simulink model "Noh_Nofusion"  (R2020b)
settings: Solver=FixedStepAuto  StartTime=0.0  StopTime=Inf  FixedStep=0.01  RelTol=1e-3
PostLoadFcn:
  | if any(exist('dsrtsu_mdlpostloadfcn', 'file') ~= 0), dsrtsu_mdlpostloadfcn('Execute', bdroot); end
InitFcn:
  | , if any(exist('rtifpga_mdlclblib', 'file') ~= 0), rtifpga_mdlclblib('Init', bdroot); end,
  | , if any(exist('dsmpb_private', 'file') ~= 0), dsmpb_private('dsmpb_mdlclblib', 'Init', bdroot); end,
undefined symbols (not defined in the file): ACC_TimeGap_DecSetSwt, ACC_TimeGap_IncSetSwt, AccelPedalPosn, AccelPedalPosnVldty, AccelPedlPosnDiagc, AccPedalOverride, ACU_ShiftInProgress, ADAS_Posn_CurLane, AESSwtReq, ALC_SwtReq, BrkPedalSts, CC_ACC_CANCEL_OFFSwt, CC_ACC_CRUISE_OFFSwt, CC_ACC_DecSetSpd_SetSwt, CC_ACC_IncSetSpd_ResuSwt, CC_ACCSwtErr, CharSpd_ms, CSA_NODE, CURRENT_GEAR, CurrentGearValid, DiscIntNeverNeededParam, DrvDoorSts, DrvSBR, DrvTrqReqOvld, ECMACCInterface, ECMRespACC, ELKSwtReq, EngLimpHomeSts, EngSpd, EngState, EngState_PHEV, EngTrqMaxActSpd, EngTrqMinAct, EPS_DrvInpTrqVal_HighReslolution, EPS_FailSts, EPS_LKATorqOvrlDlvd, EPS_LKATorqOvrlDlvdVld, EPS_LKATrqOvlDlvdSts, EPS_SteerMod, EPS_TrqSnsrSts, EQ4_APPINFO, EQ4_LA_ELEM, EQ4_LA_HDR, EQ4_LAP_ELEM, EQ4_LAP_HDR, EQ4_LH_ELEM, EQ4_LH_HDR, EQ4_LRE_ELEM, EQ4_LRE_HDR, ESS_PedSwtReq, ESS_VehSwtReq, FFogLmpSts_F_Pbox, FLWheelDriveDirection, FLWheelSpd, FrntWiprSwtSts, FrntWshrSwtSts, FRWheelDriveDirection, FRWheelSpd, HazardLmpSwtSts, HCU_AccelPedalPosn_Diag ... (+153)
libraries: simulink x132, dsmpblib x27
(part 2 of 14)

== system Noh_Nofusion/CAL ==
  Bus Assignment : BusAssignment  AssignedSignals=VehConfigHWA,VehConfigTJA,VehConfigLCK,VehConfigELK,VehConfigACC,VehConfigESS,VehConfigCC,VehConfigLKA,VehConfigLDW,VehConfigLCKIE,VehConfigiACC,VehConfigTSR,VehConfigAES
  Bus Assignment1 : BusAssignment  AssignedSignals=VehConfigADB,VehConfigHMA,VehConfigHMA_laser
  Bus Creator2 : BusCreator  Inputs=2
  Constant1 : Constant  Value=0  OutDataTypeStr=Bus: CAL_AHBC_CONFIG_BUS
  Constant2 : Constant  OutDataTypeStr=uint8
  Constant6 : Constant  Value=0  OutDataTypeStr=Bus: CAL_VSM_CONFIG_BUS
  Constant7 : Constant  OutDataTypeStr=uint8
  IfCALBus : Outport
  wires:
  Constant7/1 -> Bus Assignment/2, Bus Assignment/14, Bus Assignment/13, Bus Assignment/12, Bus Assignment/11, Bus Assignment/10, Bus Assignment/9, Bus Assignment/8, Bus Assignment/7, Bus Assignment/6, Bus Assignment/5, Bus Assignment/4, Bus Assignment/3
  Constant6/1 -> Bus Assignment/1
  Constant2/1 -> Bus Assignment1/4, Bus Assignment1/3, Bus Assignment1/2
  Bus Creator2/1 -> IfCALBus/1  "IfCALBus"
  Bus Assignment1/1 -> Bus Creator2/2  "CAL_AHBC_CONFIG"
  Bus Assignment/1 -> Bus Creator2/1  "CAL_VSM_CONFIG"
  Constant1/1 -> Bus Assignment1/1

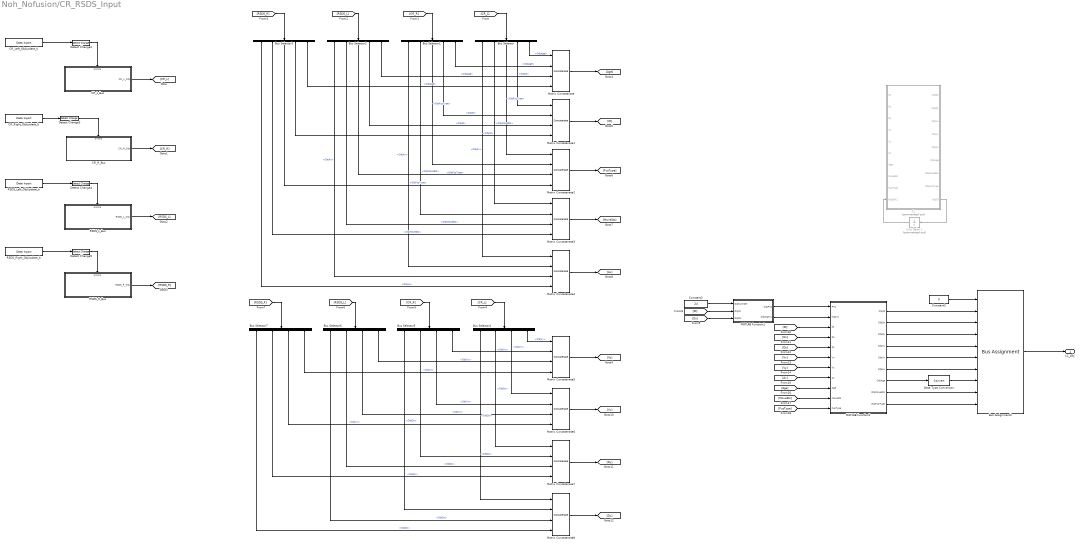
== system Noh_Nofusion/CR_RSDS_Input ==
  Bus Assignment3 : BusAssignment  AssignedSignals=Object_ID,Object_DX,Object_DY,Object_VX,Object_VY,Object_AX,Object_Age,Object_MovingState,Object_Fus_Type
  Bus Selector{,1..3} (4 alike) : BusSelector  OutputSignals=ObjAx,ObjMoveSts,ObjFusType,ObjID,ObjAge
  Bus Selector{4..7} (4 alike) : BusSelector  OutputSignals=ObjDx,ObjDy,ObjVx,ObjVy
  CL : MATLAB Function  Commented=on  TreatAsAtomicUnit=on
  CR_L_Bus : Subsystem
  CR_Left_ObjUpdate_b : dsmpblib/Data Inport  Priority=10000
      settings: SourceProductName=dSPACE Model Interface Blockset
  CR_R_Bus : Subsystem
  CR_Right_ObjUpdate_b : dsmpblib/Data Inport  Priority=10000
      settings: SourceProductName=dSPACE Model Interface Blockset
  Constant2 : Constant  Value=24  OutDataTypeStr=uint8
  Constant3 : Constant  Value=0  OutDataTypeStr=Bus: TOS_LC_BUS
  Data Type Conversion : DataTypeConversion
  Detect Change{2..5} (4 alike) : simulink/Logic and Bit Operations/Detect Change  vinit=0  OutDataTypeStr=boolean
  MATLAB Function1 : MATLAB Function  TreatAsAtomicUnit=on
  MATLAB Function2 : MATLAB Function  TreatAsAtomicUnit=on
  Matrix Concatenate{,1..8} (9 alike) : Concatenate  NumInputs=4
  RSDS_L_Bus : Subsystem
  RSDS_Left_ObjUpdate_b : dsmpblib/Data Inport  Priority=10000
      settings: SourceProductName=dSPACE Model Interface Blockset
  RSDS_R_Bus : Subsystem
  RSDS_Right_ObjUpdate_b : dsmpblib/Data Inport  Priority=10000
      settings: SourceProductName=dSPACE Model Interface Blockset
  Unit Delay1 : UnitDelay  Commented=on  SampleTime=-1  HasFrameUpgradeWarning=on
  LC_Obj : Outport  OutDataTypeStr=Bus: TOS_LC_BUS
  wires:
  Bus Selector5/4 -> Matrix Concatenate5/2  "<ObjVy>"
  [RSDS_L] -> Bus Selector2/1
  CR_Right_ObjUpdate_b/1 -> Detect Change3/1
  Matrix Concatenate8/1 -> [Dx]
  [CR_L] -> Bus Selector4/1
  Bus Selector3/5 -> Matrix Concatenate/4  "<ObjAge>"
  Bus Selector/4 -> Matrix Concatenate1/1  "<ObjID>"
  [RSDS_R] -> Bus Selector3/1
  RSDS_Left_ObjUpdate_b/1 -> Detect Change4/1
  [Vx] -> MATLAB Function2/6(Vx)
  Matrix Concatenate1/1 -> [ID]
  Bus Selector3/4 -> Matrix Concatenate1/4  "<ObjID>"
  Bus Selector1/5 -> Matrix Concatenate/2  "<ObjAge>"
  Bus Selector5/3 -> Matrix Concatenate6/2  "<ObjVx>"
  Bus Selector4/4 -> Matrix Concatenate5/1  "<ObjVy>"
  RSDS_Right_ObjUpdate_b/1 -> Detect Change5/1
  Bus Selector6/1 -> Matrix Concatenate8/3  "<ObjDx>"
  Bus Selector2/4 -> Matrix Concatenate1/3  "<ObjID>"
  Matrix Concatenate2/1 -> [FusType]
  Bus Selector7/2 -> Matrix Concatenate7/4  "<ObjDy>"
  Bus Selector2/2 -> Matrix Concatenate3/3  "<ObjMoveSts>"
  Bus Selector3/2 -> Matrix Concatenate3/4  "<ObjMoveSts>"
  Bus Selector4/1 -> Matrix Concatenate8/1  "<ObjDx>"
  Bus Selector6/2 -> Matrix Concatenate7/3  "<ObjDy>"
  Constant2/1 -> MATLAB Function1/1(ObjNumber)
  Constant3/1 -> Bus Assignment3/1
  [CR_R] -> Bus Selector5/1
  [RSDS_R] -> Bus Selector7/1
  [Dx] -> MATLAB Function2/4(Dx)
  [CR_R] -> Bus Selector1/1
  Bus Selector/5 -> Matrix Concatenate/1  "<ObjAge>"
  [FusType] -> MATLAB Function2/11(FusType)
  Bus Selector1/2 -> Matrix Concatenate3/2  "<ObjMoveSts>"
  CR_Left_ObjUpdate_b/1 -> Detect Change2/1
  Bus Selector6/4 -> Matrix Concatenate5/3  "<ObjVy>"
  Detect Change4/1 -> RSDS_L_Bus/Enable
  Detect Change5/1 -> RSDS_R_Bus/Enable
  Bus Selector/1 -> Matrix Concatenate4/1  "<ObjAx>"
  Detect Change2/1 -> CR_L_Bus/Enable
  Detect Change3/1 -> CR_R_Bus/Enable
  Bus Selector7/3 -> Matrix Concatenate6/4  "<ObjVx>"
  Bus Selector2/5 -> Matrix Concatenate/3  "<ObjAge>"
  Bus Selector3/1 -> Matrix Concatenate4/4  "<ObjAx>"
  Bus Selector7/4 -> Matrix Concatenate5/4  "<ObjVy>"
  [CR_L] -> Bus Selector/1
  MATLAB Function1/2(ObjMatrix) -> MATLAB Function2/2(Matrix)
  Bus Assignment3/1 -> LC_Obj/1
  Bus Selector6/3 -> Matrix Concatenate6/3  "<ObjVx>"
  Bus Selector2/3 -> Matrix Concatenate2/3  "<ObjFusType>"
  Matrix Concatenate3/1 -> [MoveSts]
  Matrix Concatenate7/1 -> [Dy]
  Bus Selector4/2 -> Matrix Concatenate7/1  "<ObjDy>"
  Matrix Concatenate5/1 -> [Vy]
  [Ax] -> MATLAB Function2/8(Ax)
  Bus Selector1/3 -> Matrix Concatenate2/2  "<ObjFusType>"
  Bus Selector2/1 -> Matrix Concatenate4/3  "<ObjAx>"
  [Vy] -> MATLAB Function2/7(Vy)
  Bus Selector3/3 -> Matrix Concatenate2/4  "<ObjFusType>"
  Bus Selector/3 -> Matrix Concatenate2/1  "<ObjFusType>"
  Bus Selector1/1 -> Matrix Concatenate4/2  "<ObjAx>"
  Bus Selector1/4 -> Matrix Concatenate1/2  "<ObjID>"
  Bus Selector5/2 -> Matrix Concatenate7/2  "<ObjDy>"
  [Dx] -> MATLAB Function1/3(ObjDx)
  [RSDS_L] -> Bus Selector6/1
  Bus Selector7/1 -> Matrix Concatenate8/4  "<ObjDx>"
  Bus Selector5/1 -> Matrix Concatenate8/2  "<ObjDx>"
  Bus Selector4/3 -> Matrix Concatenate6/1  "<ObjVx>"
  Bus Selector/2 -> Matrix Concatenate3/1  "<ObjMoveSts>"
  Matrix Concatenate6/1 -> [Vx]
  Matrix Concatenate4/1 -> [Ax]
  [ID] -> MATLAB Function1/2(ObjID)
  Matrix Concatenate/1 -> [Age]
  [Age] -> MATLAB Function2/9(Age)
  [Dy] -> MATLAB Function2/5(Dy)
  [MoveSts] -> MATLAB Function2/10(MoveSts)
  MATLAB Function1/1(ObjPrio) -> MATLAB Function2/1(Prio)
  [ID] -> MATLAB Function2/3(ID)
  RSDS_R_Bus/1(RSDS_R_Obj) -> [RSDS_R]
  RSDS_L_Bus/1(RSDS_L_Obj) -> [RSDS_L]
  CR_L_Bus/1(CR_L_Obj) -> [CR_L]
  CR_R_Bus/1(CR_R_Obj) -> [CR_R]
  CL/9(ObjID) -> Unit Delay1/1
  Unit Delay1/1 -> CL/10(ObjIDK1)
  MATLAB Function2/2(ObjDx) -> Bus Assignment3/3
  MATLAB Function2/1(ObjID) -> Bus Assignment3/2
  MATLAB Function2/3(ObjDy) -> Bus Assignment3/4
  MATLAB Function2/4(ObjVx) -> Bus Assignment3/5
  MATLAB Function2/5(ObjVy) -> Bus Assignment3/6
  MATLAB Function2/6(ObjAx) -> Bus Assignment3/7
  MATLAB Function2/7(ObjAge) -> Data Type Conversion/1
  MATLAB Function2/8(ObjMoveSts) -> Bus Assignment3/9
  MATLAB Function2/9(ObjFusType) -> Bus Assignment3/10
  Data Type Conversion/1 -> Bus Assignment3/8

== system Noh_Nofusion/Chassis1 ==
  note: DIAG-MON
      | (DiagnosticMonitor)
  note: HMI
      | (HumanMachineInterface)
  IfFaultTriggers : Inport
  IfFaultDTCs : Inport  Port=2
  IfVCANBus : Inport  Port=3  OutDataTypeStr=Bus: VCAN_BUS
  IfCALBus : Inport  Port=4
  IfVIEBus : Inport  Port=5
  IfVSMBus : Inport  Port=6
  IfLSMBus : Inport  Port=7
  IfLonCtrlBus : Inport  Port=8
  IfLatCtrlBus : Inport  Port=9
  IfPlanbus : Inport  Port=10
  IfVEQ4Bus : Inport  Port=11
  IfEHRBus : Inport  Port=12
  IfDMSBus : Inport  Port=13
  LaneBus : Inport  Port=14
  IfAEBBus : Inport  Port=15
  IfOSMBus : Inport  Port=16
  RoadBus : Inport  Port=17
  CSASim_IDC_L2_LampReq : Inport  Port=18
  function : TriggerPort  TriggerType=function-call  VariantControl=Variant
  Bus Assignment : BusAssignment  AssignedSignals=IFCAngCmdReqValue,IFCFuncAngCmdReqFlag,RollingCounter_IFC1,RollingCounter_IFC2
  Bus Assignment1 : BusAssignment  AssignedSignals=IFC_Line01_Dy,IFC_Line01_Curv,IFC_Line01_CurvChange,IFC_Line01_Type,IFC_Line02_Dy,IFC_Line02_Curv,IFC_Line02_CurvChange,IFC_Line02_Type,IFC_Line03_Dy,IFC_Line03_Curv,IFC_Line03_CurvChange,IFC_Line03_Type,IFC_Line04_Dy,IFC_Line04_Curv,IFC_Line04_CurvChange,IFC_Line04_Type,IFC_Roadedge01_Dy,IFC_Roadedge01_Curv,IFC_Roadedge01_CurvChange,IFC_Roadedge01_Type,IFC_Roadedge02_Dy,IFC_Roadedge02_Curv,IFC_Roadedge02_CurvChange,IFC_Roadedge02_Type
  Bus Assignment2 : BusAssignment  AssignedSignals=IFC_Line01_HeadingAngle,IFC_Line02_HeadingAngle,IFC_Line03_HeadingAngle,IFC_Line04_HeadingAngle,IFC_Roadedge01_HeadingAngle,IFC_Roadedge02_HeadingAngle
  Bus Assignment3 : BusAssignment  AssignedSignals=ACCTgtObjAx,ACCTgtObjAy,ACCTgtObjCntAlive,ACCTgtObjDx,ACCTgtObjDy,ACCTgtObjExist,ACCTgtObjID,ACCTgtObjObstcl,ACCTgtObjState,ACCTgtObjVideoCfmd,ACCTgtObjVx,ACCTgtObjVy,ACC_SOSReq,BrdgDst,CurveDst,DrvgOnHiWay,DrvgOnRiLane,DrvrSts,HandsoffDetd,MapDataValid,NavSpdLimUnit,RampDst,RoadCrvt,RoadCrvtFar,SpdLimit,SpdLimitDst,TunnelDst
  Bus Assignment4 : BusAssignment  AssignedSignals=Longctrl_DecelToStopReq,Longctrl_Decel_Req,Longctrl_Decel_ReqValue,Longctrl_EngTrqReq,Longctrl_EngTrqReqActive,Longctrl_HCUTrqReq,Longctrl_HCUTrqReqActive,ACC_CRInterface,ActualTargetSpeed,Longctrl_DrvOFF_Req,Longctrl_FuelCutOffPrevn,Longctrl_ModSts,Longctrl_ParkShiftReq,Longctrl_VehHldReq,HWP_TgtAccel_L2,RollingCounter_ACC1,RollingCounter_ACC2,RollingCounter_ACC10
  Bus Assignment5 : BusAssignment  AssignedSignals=ACC_EgoStatus,ACC_FctSts,ACC_InterSysInfoDisp,ACC_LeTargrtDection,ACC_LeTargrt_02_Detn,ACC_LeTgtDx,ACC_LeTgtDy,ACC_LeTgtHeading,ACC_LeTgtObjBarDisp,ACC_LeTgtTyp,ACC_LeTgt_02_Dx,ACC_LeTgt_02_Dy,ACC_LeTgt_02_Typ,ACC_LeTgtfusion,ACC_ModDisp,ACC_ObjDetecte,ACC_PotentialTgtDetn,ACC_PotentialTgtDx,ACC_PotentialTgtDy,ACC_PotentialTgtHeading,ACC_PotentialTgtTyp,ACC_PotentialTgtfusion,ACC_RiTargrtDetn,ACC_RiTargrt_02_Detn,ACC_RiTgtDx,ACC_RiTgtDy,ACC_RiTgtHeading,ACC_RiTgtObjBarDisp,ACC_RiTgtTyp,ACC_RiTgt_02_Dx,ACC_RiTgt_02_Dy,ACC_RiTgt_02_Typ,ACC_RiTgtfusion,ACC_RlvTgtDetn,ACC_RlvTgtDx,ACC_RlvTgtDy,ACC_RlvTgtHeading,ACC_RlvTgtTyp,ACC_RlvTgtfusion,ACC_SpdSetValue,ACC_TakeOverReq,ACC_TgtObjBarDisp,ACC_TimeGapSet,ADAS_DriverInloop_Monitor,ALC_InterSysInfoDisp,ALC_Resp,CruCha_ModDisp,CruChar_InterSysInfoDisp,HWA_InterSysInfoDisp,HWA_LaneChange,HWA_LaneChangeReq,HWA_ModDisp,HWA_Resp,HWA_SnvtySet_Resp,HWA_warning,ICA_HandsOffResp,ISL_InterSysInfoDisp,ISL_Resp,IntelligentCurveAct,Request_driveoff,TJA_ACC_SelSts,TJA_ICA_InterSysInfoDisp,TJA_ICA_ModDisp,RollingCounter_ACC3,RollingCounter_ACC4,RollingCounter_ACC8,RollingCounter_ACC6,RollingCounter_ACC7
  Bus Assignment6 : BusAssignment  AssignedSignals=AESErrSts,AESResp,AESSts,AESintervention,CameraBlockageSts,ELKMainState,ELKResp,ESSErrSts,ESSSts,ESS_PedResp,ESS_VehResp,ESSintervention,IFCCalibrationSts,IFCHUTInterface,IFC_Handsoffwarn,IFC_LaneCurve,IFC_LeLaneTyp,IFC_LeLane_dy,IFC_NextLeLaneTyp,IFC_NextLeLane_dy,IFC_NextRiLaneTyp,IFC_NextRiLane_dy,IFC_RiLaneTyp,IFC_RiLane_dy,IntelligentEvaResp,LCKResp,LDWResp,LDW_LKAWarn,LDW_LKA_Snvty,LKAResp,LSSErrSts,LSSFuncSts,LSSIntervention,LSSResp,LSSWarnFormResp,LaneAvailability,TJA_FollowSts,RollingCounter_IFC3,RollingCounter_IFC4,RollingCounter_IFC5,RollingCounter_IFC6
  Bus Assignment7 : BusAssignment  AssignedSignals=IDC_L2_EmgyLightReq,IDC_L2_FWiperReq,IDC_L2_TurnLightReq,RollingCounter_IFC7
  Bus Selector : BusSelector  OutputSignals=LONC_CTRL_OUT.Longctrl_Decel_Req,LONC_CTRL_OUT.Longctrl_Decel_ReqValue,LONC_CTRL_OUT.Longctrl_EngTrqReq,LONC_CTRL_OUT.Longctrl_EngTrqReqActive,LONC_Hybrid_CTRL_OUT.Longctrl_HCUTrqReq,LONC_Hybrid_CTRL_OUT.Longctrl_HCUTrqReqActive
  Bus Selector1 : BusSelector  OutputSignals=LATC_IFCAngCmdReqValue,LATC_IFCFuncAngCmdReqFlag
  Bus Selector10 : BusSelector  OutputSignals=HMI_ACC_FD4.ACCTgtObjAx,HMI_ACC_FD4.ACCTgtObjAy,HMI_ACC_FD4.ACCTgtObjCntAlive,HMI_ACC_FD4.ACCTgtObjDx,HMI_ACC_FD4.ACCTgtObjDy,HMI_ACC_FD4.ACCTgtObjExist,HMI_ACC_FD4.ACCTgtObjID,HMI_ACC_FD4.ACCTgtObjObstcl,HMI_ACC_FD4.ACCTgtObjState,HMI_ACC_FD4.ACCTgtObjVideoCfmd,HMI_ACC_FD4.ACCTgtObjVx,HMI_ACC_FD4.ACCTgtObjVy,HMI_ACC_FD4.ACC_SOSReq,HMI_ACC_FD4.BrdgDst,HMI_ACC_FD4.CurveDst,HMI_ACC_FD4.DrvgOnHiWay,HMI_ACC_FD4.DrvgOnRiLane,HMI_ACC_FD4.DrvrSts,HMI_ACC_FD4.HandsoffDetd,HMI_ACC_FD4.MapDataValid,HMI_ACC_FD4.NavSpdLimUnit,HMI_ACC_FD4.RampDst,HMI_ACC_FD4.RoadCrvt,HMI_ACC_FD4.RoadCrvtFar,HMI_ACC_FD4.SpdLimit,HMI_ACC_FD4.SpdLimitDst,HMI_ACC_FD4.TunnelDst
  Bus Selector18 : BusSelector  OutputSignals=PLAN_Longctrl_DecelToStopReq
  Bus Selector19 : BusSelector  OutputSignals=HMI_IFC_FD3.IDC_L2_EmgyLightReq,HMI_IFC_FD3.IDC_L2_FWiperReq
  Bus Selector2 : BusSelector  OutputSignals=HMI_ACC_FD1.ACC_CRInterface,HMI_ACC_FD1.ActualTargetSpeed,HMI_ACC_FD1.Longctrl_DrvOFF_Req,HMI_ACC_FD1.Longctrl_FuelCutOffPrevn,HMI_ACC_FD1.Longctrl_ModSts,HMI_ACC_FD1.Longctrl_ParkShiftReq,HMI_ACC_FD1.Longctrl_VehHldReq
  Bus Selector3 : BusSelector  OutputSignals=AESErrSts,HMI_IFC_FD2.AESResp,HMI_IFC_FD2.AESSts,HMI_IFC_FD2.AESintervention,HMI_IFC_FD2.CameraBlockageSts,HMI_IFC_FD2.ELKMainState,HMI_IFC_FD2.ELKResp,ESSErrSts,HMI_IFC_FD2.ESSSts,HMI_IFC_FD2.ESS_PedResp,HMI_IFC_FD2.ESS_VehResp,HMI_IFC_FD2.ESSintervention,HMI_IFC_FD2.IFCCalibrationSts,HMI_IFC_FD2.IFCHUTInterface,HMI_IFC_FD2.IFC_Handsoffwarn,HMI_IFC_FD2.IFC_LaneCurve,HMI_IFC_FD2.IFC_LeLaneTyp,HMI_IFC_FD2.IFC_LeLane_dy,HMI_IFC_FD2.IFC_NextLeLaneTyp,HMI_IFC_FD2.IFC_NextLeLane_dy,HMI_IFC_FD2.IFC_NextRiLaneTyp,HMI_IFC_FD2.IFC_NextRiLane_dy,HMI_IFC_FD2.IFC_RiLaneTyp,HMI_IFC_FD2.IFC_RiLane_dy,HMI_IFC_FD2.IntelligentEvaResp,HMI_IFC_FD2.LCKResp,HMI_IFC_FD2.LDWResp,HMI_IFC_FD2.LDW_LKAWarn,HMI_IFC_FD2.LDW_LKA_Snvty,HMI_IFC_FD2.LKAResp,HMI_IFC_FD2.LSSErrSts,HMI_IFC_FD2.LSSFuncSts,HMI_IFC_FD2.LSSIntervention,HMI_IFC_FD2.LSSResp,HMI_IFC_FD2.LSSWarnFormResp,HMI_IFC_FD2.LaneAvailability,HMI_IFC_FD2.TJA_FollowSts
  Bus Selector5 : BusSelector  OutputSignals=HMI_IFC_FD5.IFC_Line01_Dy,HMI_IFC_FD5.IFC_Line01_Curv,HMI_IFC_FD5.IFC_Line01_CurvChange,HMI_IFC_FD5.IFC_Line01_Type,HMI_IFC_FD5.IFC_Line02_Dy,HMI_IFC_FD5.IFC_Line02_Curv,HMI_IFC_FD5.IFC_Line02_CurvChange,HMI_IFC_FD5.IFC_Line02_Type,HMI_IFC_FD5.IFC_Line03_Dy,HMI_IFC_FD5.IFC_Line03_Curv,HMI_IFC_FD5.IFC_Line03_CurvChange,HMI_IFC_FD5.IFC_Line03_Type,HMI_IFC_FD5.IFC_Line04_Dy,HMI_IFC_FD5.IFC_Line04_Curv,HMI_IFC_FD5.IFC_Line04_CurvChange,HMI_IFC_FD5.IFC_Line04_Type,HMI_IFC_FD5.IFC_Roadedge01_Dy,HMI_IFC_FD5.IFC_Roadedge01_Curv,HMI_IFC_FD5.IFC_Roadedge01_CurvChange,HMI_IFC_FD5.IFC_Roadedge01_Type,HMI_IFC_FD5.IFC_Roadedge02_Dy,HMI_IFC_FD5.IFC_Roadedge02_Curv,HMI_IFC_FD5.IFC_Roadedge02_CurvChange,HMI_IFC_FD5.IFC_Roadedge02_Type
  Bus Selector6 : BusSelector  OutputSignals=HMI_IFC_FD6.IFC_Line01_HeadingAngle,HMI_IFC_FD6.IFC_Line02_HeadingAngle,HMI_IFC_FD6.IFC_Line03_HeadingAngle,HMI_IFC_FD6.IFC_Line04_HeadingAngle,HMI_IFC_FD6.IFC_Roadedge01_HeadingAngle,HMI_IFC_FD6.IFC_Roadedge02_HeadingAngle
  Bus Selector8 : BusSelector  OutputSignals=HMI_ACC_FD2.ACC_EgoStatus,HMI_ACC_FD2.ACC_FctSts,HMI_ACC_FD2.ACC_InterSysInfoDisp,HMI_ACC_FD2.ACC_LeTargrtDection,HMI_ACC_FD2.ACC_LeTargrt_02_Detn,HMI_ACC_FD2.ACC_LeTgtDx,HMI_ACC_FD2.ACC_LeTgtDy,HMI_ACC_FD2.ACC_LeTgtHeading,HMI_ACC_FD2.ACC_LeTgtObjBarDisp,HMI_ACC_FD2.ACC_LeTgtTyp,HMI_ACC_FD2.ACC_LeTgt_02_Dy,HMI_ACC_FD2.ACC_LeTgt_02_Dx,HMI_ACC_FD2.ACC_LeTgt_02_Typ,HMI_ACC_FD2.ACC_LeTgtfusion,HMI_ACC_FD2.ACC_ModDisp,HMI_ACC_FD2.ACC_ObjDetecte,HMI_ACC_FD2.ACC_PotentialTgtDetn,HMI_ACC_FD2.ACC_PotentialTgtDx,HMI_ACC_FD2.ACC_PotentialTgtDy,HMI_ACC_FD2.ACC_PotentialTgtHeading,HMI_ACC_FD2.ACC_PotentialTgtTyp,HMI_ACC_FD2.ACC_PotentialTgtfusion,HMI_ACC_FD2.ACC_RiTargrtDetn,HMI_ACC_FD2.ACC_RiTargrt_02_Detn,HMI_ACC_FD2.ACC_RiTgtDx,HMI_ACC_FD2.ACC_RiTgtDy,HMI_ACC_FD2.ACC_RiTgtHeading,HMI_ACC_FD2.ACC_RiTgtObjBarDisp,HMI_ACC_FD2.ACC_RiTgtTyp,HMI_ACC_FD2.ACC_RiTgt_02_Dx,HMI_ACC_FD2.ACC_RiTgt_02_Dy,HMI_ACC_FD2.ACC_RiTgt_02_Typ,HMI_ACC_FD2.ACC_RiTgtfusion,HMI_ACC_FD2.ACC_RlvTgtDetn,HMI_ACC_FD2.ACC_RlvTgtDx,HMI_ACC_FD2.ACC_RlvTgtDy,HMI_ACC_FD2.ACC_RlvTgtHeading,HMI_ACC_FD2.ACC_RlvTgtTyp,HMI_ACC_FD2.ACC_RlvTgtfusion,HMI_ACC_FD2.ACC_SpdSetValue,HMI_ACC_FD2.ACC_TakeOverReq,HMI_ACC_FD2.ACC_TgtObjBarDisp,HMI_ACC_FD2.ACC_TimeGapSet,HMI_ACC_FD2.ADAS_DriverInloop_Monitor,HMI_ACC_FD2.ALC_InterSysInfoDisp,HMI_ACC_FD2.ALC_Resp,HMI_ACC_FD2.CruCha_ModDisp,HMI_ACC_FD2.CruChar_InterSysInfoDisp,HMI_ACC_FD2.HWA_InterSysInfoDisp,HMI_ACC_FD2.HWA_LaneChange,HMI_ACC_FD2.HWA_LaneChangeReq,HMI_ACC_FD2.HWA_ModDisp,HMI_ACC_FD2.HWA_Resp,HMI_ACC_FD2.HWA_SnvtySet_Resp,HMI_ACC_FD2.HWA_warning,HMI_ACC_FD2.ICA_HandsOffResp,HMI_ACC_FD2.ISL_InterSysInfoDisp,HMI_ACC_FD2.ISL_Resp,HMI_ACC_FD2.IntelligentCurveAct,HMI_ACC_FD2.Request_driveoff,HMI_ACC_FD2.TJA_ACC_SelSts,HMI_ACC_FD2.TJA_ICA_InterSysInfoDisp,HMI_ACC_FD2.TJA_ICA_ModDisp
  Constant : Constant  Value=0  OutDataTypeStr=Bus: IFC_FD1_MSG_BUS
  Constant10 : Constant  Value=0  OutDataTypeStr=Bus: ACC_FD2_MSG_BUS
  Constant12 : Constant  Value=0  OutDataTypeStr=Bus: IFC_FD3_MSG_BUS
  Constant3 : Constant  Value=0  OutDataTypeStr=Bus: IFC_FD2_MSG_BUS
  Constant5 : Constant  Value=0  OutDataTypeStr=Bus: IFC_FD5_MSG_BUS
  Constant6 : Constant  Value=0  OutDataTypeStr=Bus: IFC_FD6_MSG_BUS
  Constant7 : Constant  Value=0  OutDataTypeStr=Bus: ACC_FD4_MSG_BUS
  Constant8 : Constant  Value=0  OutDataTypeStr=Bus: ACC_FD1_MSG_BUS
  Constant9 : Constant  Value=127  OutDataTypeStr=int8
  Counter Limited{,1..4} (5 alike) : simulink/Sources/Counter Limited  uplimit=15  tsamp=-1
  HMA : Subsystem  Commented=on
  HMI : Subsystem
  IfPlanbus1 : InportShadow  Port=10
  IFC_FD1 : Outport
  IFC_FD2 : Outport  Port=2
  IFC_FD3 : Outport  Port=3
  IFC_FD5 : Outport  Port=4
  IFC_FD6 : Outport  Port=5
  ACC_FD1 : Outport  Port=6
  ACC_FD2 : Outport  Port=7
  ACC_FD4 : Outport  Port=8
  wires:
  IfVCANBus/1 -> HMI/1(IfVCANBus), HMA/1(IfCANBus)
  IfVEQ4Bus/1 -> HMA/4(IfEQ4Bus)
  IfCALBus/1 -> HMA/2(IfCALBus)
  IfFaultTriggers/1 -> HMA/3(IfDIAGBus), HMI/2(IfFaultTriggers)
  IfLonCtrlBus/1 -> [IfLonCtrlBus], HMI/5(IfLonCtrlBus)  "IfLonCtrlBus"
  IfOSMBus/1 -> HMI/6(IfOSMBus)
  IfAEBBus/1 -> HMI/7(IfAEBBus)
  IfEHRBus/1 -> HMI/8(IfEHRBus)
  IfDMSBus/1 -> HMI/9(IfDMSBus)
  LaneBus/1 -> HMI/10(LaneBus)
  RoadBus/1 -> HMI/11(RoadBus)
  HMI/1(IfHMIBus) -> Bus Selector2/1, Bus Selector10/1, Bus Selector8/1, Bus Selector6/1, Bus Selector5/1, Bus Selector19/1, Bus Selector3/1  "HMI"
  IfVSMBus/1 -> [IfVSMBus], HMI/4(IfVSMBus)
  Bus Assignment3/1 -> ACC_FD4/1
  Bus Assignment4/1 -> ACC_FD1/1
  IfPlanbus/1 -> HMI/3(IfPlanbus)
  IfPlanbus1/1 -> Bus Selector18/1
  Bus Selector18/1 -> Bus Assignment4/2  "<PLAN_Longctrl_DecelToStopReq>"
  Bus Selector1/1 -> Bus Assignment/2  "<LATC_IFCAngCmdReqValue>"
  Bus Selector1/2 -> Bus Assignment/3  "<LATC_IFCFuncAngCmdReqFlag>"
  IfLatCtrlBus/1 -> Bus Selector1/1
  Constant/1 -> Bus Assignment/1
  Bus Assignment/1 -> IFC_FD1/1
  Constant5/1 -> Bus Assignment1/1
  Bus Selector5/1 -> Bus Assignment1/2  "<IFC_Line01_Dy>"
  Bus Selector5/2 -> Bus Assignment1/3  "<IFC_Line01_Curv>"
  Bus Selector5/3 -> Bus Assignment1/4  "<IFC_Line01_CurvChange>"
  Bus Selector5/4 -> Bus Assignment1/5  "<IFC_Line01_Type>"
  Bus Selector5/5 -> Bus Assignment1/6  "<IFC_Line02_Dy>"
  Bus Selector5/6 -> Bus Assignment1/7  "<IFC_Line02_Curv>"
  Bus Selector5/7 -> Bus Assignment1/8  "<IFC_Line02_CurvChange>"
  Bus Selector5/8 -> Bus Assignment1/9  "<IFC_Line02_Type>"
  Bus Selector5/9 -> Bus Assignment1/10  "<IFC_Line03_Dy>"
  Bus Selector5/10 -> Bus Assignment1/11  "<IFC_Line03_Curv>"
  Bus Selector5/11 -> Bus Assignment1/12  "<IFC_Line03_CurvChange>"
  Bus Selector5/12 -> Bus Assignment1/13  "<IFC_Line03_Type>"
  Bus Selector5/13 -> Bus Assignment1/14  "<IFC_Line04_Dy>"
  Bus Selector5/14 -> Bus Assignment1/15  "<IFC_Line04_Curv>"
  Bus Selector5/15 -> Bus Assignment1/16  "<IFC_Line04_CurvChange>"
  Bus Selector5/16 -> Bus Assignment1/17  "<IFC_Line04_Type>"
  Bus Selector5/17 -> Bus Assignment1/18  "<IFC_Roadedge01_Dy>"
  Bus Selector5/18 -> Bus Assignment1/19  "<IFC_Roadedge01_Curv>"
  Bus Selector5/19 -> Bus Assignment1/20  "<IFC_Roadedge01_CurvChange>"
  Bus Selector5/20 -> Bus Assignment1/21  "<IFC_Roadedge01_Type>"
  Bus Selector5/21 -> Bus Assignment1/22  "<IFC_Roadedge02_Dy>"
  Bus Selector5/22 -> Bus Assignment1/23  "<IFC_Roadedge02_Curv>"
  Bus Selector5/23 -> Bus Assignment1/24  "<IFC_Roadedge02_CurvChange>"
  Bus Selector5/24 -> Bus Assignment1/25  "<IFC_Roadedge02_Type>"
  Bus Assignment1/1 -> IFC_FD5/1
  Constant6/1 -> Bus Assignment2/1
  Bus Selector6/6 -> Bus Assignment2/7  "<IFC_Roadedge02_HeadingAngle>"
  Bus Selector6/5 -> Bus Assignment2/6  "<IFC_Roadedge01_HeadingAngle>"
  Bus Selector6/4 -> Bus Assignment2/5  "<IFC_Line04_HeadingAngle>"
  Bus Selector6/3 -> Bus Assignment2/4  "<IFC_Line03_HeadingAngle>"
  Bus Selector6/2 -> Bus Assignment2/3  "<IFC_Line02_HeadingAngle>"
  Bus Selector6/1 -> Bus Assignment2/2  "<IFC_Line01_HeadingAngle>"
  Bus Assignment2/1 -> IFC_FD6/1
  Constant7/1 -> Bus Assignment3/1
  Bus Selector10/1 -> Bus Assignment3/2  "<ACCTgtObjAx>"
  Bus Selector10/2 -> Bus Assignment3/3  "<ACCTgtObjAy>"
  Bus Selector10/3 -> Bus Assignment3/4  "<ACCTgtObjCntAlive>"
  Bus Selector10/4 -> Bus Assignment3/5  "<ACCTgtObjDx>"
  Bus Selector10/5 -> Bus Assignment3/6  "<ACCTgtObjDy>"
  Bus Selector10/6 -> Bus Assignment3/7  "<ACCTgtObjExist>"
  Bus Selector10/7 -> Bus Assignment3/8  "<ACCTgtObjID>"
  Bus Selector10/8 -> Bus Assignment3/9  "<ACCTgtObjObstcl>"
  Bus Selector10/9 -> Bus Assignment3/10  "<ACCTgtObjState>"
  Bus Selector10/10 -> Bus Assignment3/11  "<ACCTgtObjVideoCfmd>"
  Bus Selector10/11 -> Bus Assignment3/12  "<ACCTgtObjVx>"
  Bus Selector10/12 -> Bus Assignment3/13  "<ACCTgtObjVy>"
  Bus Selector10/13 -> Bus Assignment3/14  "<ACC_SOSReq>"
  Bus Selector10/14 -> Bus Assignment3/15  "<BrdgDst>"
  Bus Selector10/15 -> Bus Assignment3/16  "<CurveDst>"
  Bus Selector10/16 -> Bus Assignment3/17  "<DrvgOnHiWay>"
  Bus Selector10/17 -> Bus Assignment3/18  "<DrvgOnRiLane>"
  Bus Selector10/18 -> Bus Assignment3/19  "<DrvrSts>"
  Bus Selector10/19 -> Bus Assignment3/20  "<HandsoffDetd>"
  Bus Selector10/20 -> Bus Assignment3/21  "<MapDataValid>"
  Bus Selector10/21 -> Bus Assignment3/22  "<NavSpdLimUnit>"
  Bus Selector10/22 -> Bus Assignment3/23  "<RampDst>"
  Bus Selector10/23 -> Bus Assignment3/24  "<RoadCrvt>"
  Bus Selector10/24 -> Bus Assignment3/25  "<RoadCrvtFar>"
  Bus Selector10/25 -> Bus Assignment3/26  "<SpdLimit>"
  Bus Selector10/26 -> Bus Assignment3/27  "<SpdLimitDst>"
  Bus Selector10/27 -> Bus Assignment3/28  "<TunnelDst>"
  Constant9/1 -> Bus Assignment4/16
  Bus Selector2/7 -> Bus Assignment4/15  "<Longctrl_VehHldReq>"
  Bus Selector2/6 -> Bus Assignment4/14  "<Longctrl_ParkShiftReq>"
  Bus Selector2/5 -> Bus Assignment4/13  "<Longctrl_ModSts>"
  Bus Selector2/4 -> Bus Assignment4/12  "<Longctrl_FuelCutOffPrevn>"
  Bus Selector2/3 -> Bus Assignment4/11  "<Longctrl_DrvOFF_Req>"
  Bus Selector2/2 -> Bus Assignment4/10  "<ActualTargetSpeed>"
  Bus Selector2/1 -> Bus Assignment4/9  "<ACC_CRInterface>"
  Constant8/1 -> Bus Assignment4/1
  Counter Limited/1 -> Bus Assignment4/18, Bus Assignment4/17, Bus Assignment4/19
  [IfLonCtrlBus] -> Bus Selector/1
  Bus Selector/3 -> Bus Assignment4/5  "<Longctrl_EngTrqReq>"
  Bus Selector/2 -> Bus Assignment4/4  "<Longctrl_Decel_ReqValue>"
  Bus Selector/4 -> Bus Assignment4/6  "<Longctrl_EngTrqReqActive>"
  Bus Selector/1 -> Bus Assignment4/3  "<Longctrl_Decel_Req>"
  Bus Selector/5 -> Bus Assignment4/7  "<Longctrl_HCUTrqReq>"
  Bus Selector/6 -> Bus Assignment4/8  "<Longctrl_HCUTrqReqActive>"
  Constant10/1 -> Bus Assignment5/1
  Bus Selector8/1 -> Bus Assignment5/2  "<ACC_EgoStatus>"
  Bus Selector8/2 -> Bus Assignment5/3  "<ACC_FctSts>"
  Bus Selector8/3 -> Bus Assignment5/4  "<ACC_InterSysInfoDisp>"
  Bus Selector8/4 -> Bus Assignment5/5  "<ACC_LeTargrtDection>"
  Bus Selector8/5 -> Bus Assignment5/6  "<ACC_LeTargrt_02_Detn>"
  Bus Selector8/6 -> Bus Assignment5/7  "<ACC_LeTgtDx>"
  Bus Selector8/7 -> Bus Assignment5/8  "<ACC_LeTgtDy>"
  Bus Selector8/8 -> Bus Assignment5/9  "<ACC_LeTgtHeading>"
  Bus Selector8/9 -> Bus Assignment5/10  "<ACC_LeTgtObjBarDisp>"
  Bus Selector8/10 -> Bus Assignment5/11  "<ACC_LeTgtTyp>"
  Bus Selector8/11 -> Bus Assignment5/12  "<ACC_LeTgt_02_Dy>"
  Bus Selector8/12 -> Bus Assignment5/13  "<ACC_LeTgt_02_Dx>"
  Bus Selector8/13 -> Bus Assignment5/14  "<ACC_LeTgt_02_Typ>"
  Bus Selector8/14 -> Bus Assignment5/15  "<ACC_LeTgtfusion>"
  Bus Selector8/15 -> Bus Assignment5/16  "<ACC_ModDisp>"
  Bus Selector8/16 -> Bus Assignment5/17  "<ACC_ObjDetecte>"
  Bus Selector8/17 -> Bus Assignment5/18  "<ACC_PotentialTgtDetn>"
  Bus Selector8/18 -> Bus Assignment5/19  "<ACC_PotentialTgtDx>"
  Bus Selector8/19 -> Bus Assignment5/20  "<ACC_PotentialTgtDy>"
  Bus Selector8/20 -> Bus Assignment5/21  "<ACC_PotentialTgtHeading>"
  Bus Selector8/21 -> Bus Assignment5/22  "<ACC_PotentialTgtTyp>"
  Bus Selector8/22 -> Bus Assignment5/23  "<ACC_PotentialTgtfusion>"
  Bus Selector8/23 -> Bus Assignment5/24  "<ACC_RiTargrtDetn>"
  Bus Selector8/24 -> Bus Assignment5/25  "<ACC_RiTargrt_02_Detn>"
  Bus Selector8/25 -> Bus Assignment5/26  "<ACC_RiTgtDx>"
  Bus Selector8/26 -> Bus Assignment5/27  "<ACC_RiTgtDy>"
  Bus Selector8/27 -> Bus Assignment5/28  "<ACC_RiTgtHeading>"
  Bus Selector8/28 -> Bus Assignment5/29  "<ACC_RiTgtObjBarDisp>"
  Bus Selector8/29 -> Bus Assignment5/30  "<ACC_RiTgtTyp>"
  Bus Selector8/30 -> Bus Assignment5/31  "<ACC_RiTgt_02_Dx>"
  Bus Selector8/31 -> Bus Assignment5/32  "<ACC_RiTgt_02_Dy>"
  Bus Selector8/32 -> Bus Assignment5/33  "<ACC_RiTgt_02_Typ>"
  Bus Selector8/33 -> Bus Assignment5/34  "<ACC_RiTgtfusion>"
  Bus Selector8/34 -> Bus Assignment5/35  "<ACC_RlvTgtDetn>"
  Bus Selector8/35 -> Bus Assignment5/36  "<ACC_RlvTgtDx>"
  Bus Selector8/36 -> Bus Assignment5/37  "<ACC_RlvTgtDy>"
  Bus Selector8/37 -> Bus Assignment5/38  "<ACC_RlvTgtHeading>"
  Bus Selector8/38 -> Bus Assignment5/39  "<ACC_RlvTgtTyp>"
  Bus Selector8/39 -> Bus Assignment5/40  "<ACC_RlvTgtfusion>"
  Bus Selector8/40 -> Bus Assignment5/41  "<ACC_SpdSetValue>"
  Bus Selector8/41 -> Bus Assignment5/42  "<ACC_TakeOverReq>"
  Bus Selector8/42 -> Bus Assignment5/43  "<ACC_TgtObjBarDisp>"
  Bus Selector8/43 -> Bus Assignment5/44  "<ACC_TimeGapSet>"
  Bus Selector8/44 -> Bus Assignment5/45  "<ADAS_DriverInloop_Monitor>"
  Bus Selector8/45 -> Bus Assignment5/46  "<ALC_InterSysInfoDisp>"
  Bus Selector8/46 -> Bus Assignment5/47  "<ALC_Resp>"
  Bus Selector8/47 -> Bus Assignment5/48  "<CruCha_ModDisp>"
  Bus Selector8/48 -> Bus Assignment5/49  "<CruChar_InterSysInfoDisp>"
  Bus Selector8/49 -> Bus Assignment5/50  "<HWA_InterSysInfoDisp>"
  Bus Selector8/50 -> Bus Assignment5/51  "<HWA_LaneChange>"
  Bus Selector8/51 -> Bus Assignment5/52  "<HWA_LaneChangeReq>"
  Bus Selector8/52 -> Bus Assignment5/53  "<HWA_ModDisp>"
  Bus Selector8/53 -> Bus Assignment5/54  "<HWA_Resp>"
  Bus Selector8/54 -> Bus Assignment5/55  "<HWA_SnvtySet_Resp>"
  Bus Selector8/55 -> Bus Assignment5/56  "<HWA_warning>"
  Bus Selector8/56 -> Bus Assignment5/57  "<ICA_HandsOffResp>"
  Bus Selector8/57 -> Bus Assignment5/58  "<ISL_InterSysInfoDisp>"
  Bus Selector8/58 -> Bus Assignment5/59  "<ISL_Resp>"
  Bus Selector8/59 -> Bus Assignment5/60  "<IntelligentCurveAct>"
  Counter Limited1/1 -> Bus Assignment5/68, Bus Assignment5/65, Bus Assignment5/66, Bus Assignment5/67, Bus Assignment5/69
  Bus Selector8/60 -> Bus Assignment5/61  "<Request_driveoff>"
  Bus Selector8/61 -> Bus Assignment5/62  "<TJA_ACC_SelSts>"
  Bus Selector8/62 -> Bus Assignment5/63  "<TJA_ICA_InterSysInfoDisp>"
  Bus Selector8/63 -> Bus Assignment5/64  "<TJA_ICA_ModDisp>"
  Bus Assignment5/1 -> ACC_FD2/1
  Constant3/1 -> Bus Assignment6/1
  Bus Selector3/1 -> Bus Assignment6/2  "<AESErrSts>"
  Bus Selector3/2 -> Bus Assignment6/3  "<AESResp>"
  Bus Selector3/3 -> Bus Assignment6/4  "<AESSts>"
  Bus Selector3/4 -> Bus Assignment6/5  "<AESintervention>"
  Bus Selector3/5 -> Bus Assignment6/6  "<CameraBlockageSts>"
  Bus Selector3/6 -> Bus Assignment6/7  "<ELKMainState>"
  Bus Selector3/7 -> Bus Assignment6/8  "<ELKResp>"
  Bus Selector3/8 -> Bus Assignment6/9  "<ESSErrSts>"
  Bus Selector3/9 -> Bus Assignment6/10  "<ESSSts>"
  Bus Selector3/10 -> Bus Assignment6/11  "<ESS_PedResp>"
  Bus Selector3/11 -> Bus Assignment6/12  "<ESS_VehResp>"
  Bus Selector3/12 -> Bus Assignment6/13  "<ESSintervention>"
  Bus Selector3/13 -> Bus Assignment6/14  "<IFCCalibrationSts>"
  Bus Selector3/14 -> Bus Assignment6/15  "<IFCHUTInterface>"
  Bus Selector3/15 -> Bus Assignment6/16  "<IFC_Handsoffwarn>"
  Bus Selector3/16 -> Bus Assignment6/17  "<IFC_LaneCurve>"
  Bus Selector3/17 -> Bus Assignment6/18  "<IFC_LeLaneTyp>"
  Bus Selector3/18 -> Bus Assignment6/19  "<IFC_LeLane_dy>"
  Bus Selector3/19 -> Bus Assignment6/20  "<IFC_NextLeLaneTyp>"
  Bus Selector3/20 -> Bus Assignment6/21  "<IFC_NextLeLane_dy>"
  Bus Selector3/21 -> Bus Assignment6/22  "<IFC_NextRiLaneTyp>"
  Bus Selector3/22 -> Bus Assignment6/23  "<IFC_NextRiLane_dy>"
  Bus Selector3/23 -> Bus Assignment6/24  "<IFC_RiLaneTyp>"
  Bus Selector3/24 -> Bus Assignment6/25  "<IFC_RiLane_dy>"
  Bus Selector3/25 -> Bus Assignment6/26  "<IntelligentEvaResp>"
  Bus Selector3/26 -> Bus Assignment6/27  "<LCKResp>"
  Bus Selector3/27 -> Bus Assignment6/28  "<LDWResp>"
  Bus Selector3/28 -> Bus Assignment6/29  "<LDW_LKAWarn>"
  Bus Selector3/29 -> Bus Assignment6/30  "<LDW_LKA_Snvty>"
  Bus Selector3/30 -> Bus Assignment6/31  "<LKAResp>"
  Bus Selector3/31 -> Bus Assignment6/32  "<LSSErrSts>"
  Bus Selector3/32 -> Bus Assignment6/33  "<LSSFuncSts>"
  Bus Selector3/33 -> Bus Assignment6/34  "<LSSIntervention>"
  Bus Selector3/34 -> Bus Assignment6/35  "<LSSResp>"
  Bus Selector3/35 -> Bus Assignment6/36  "<LSSWarnFormResp>"
  Bus Selector3/36 -> Bus Assignment6/37  "<LaneAvailability>"
  Bus Selector3/37 -> Bus Assignment6/38  "<TJA_FollowSts>"
  Counter Limited2/1 -> Bus Assignment6/40, Bus Assignment6/39, Bus Assignment6/41, Bus Assignment6/42
  Bus Assignment6/1 -> IFC_FD2/1
  Counter Limited3/1 -> Bus Assignment/4, Bus Assignment/5
  Constant12/1 -> Bus Assignment7/1
  Bus Selector19/1 -> Bus Assignment7/2  "<IDC_L2_EmgyLightReq>"
  Bus Selector19/2 -> Bus Assignment7/3  "<IDC_L2_FWiperReq>"
  Counter Limited4/1 -> Bus Assignment7/5
  Bus Assignment7/1 -> IFC_FD3/1
  CSASim_IDC_L2_LampReq/1 -> Bus Assignment7/4

== system Noh_Nofusion/Common1 ==
  note: EHR
      | (ElectronicHorizonReconstructor)
  note: DMS
      | (DriverMonitorSystem)
  note: CAL
      | (ConfigurationCalibration)
  note: VIE
      | (VehicleInfomationEvaluation)
  IfCANBus : Inport
  function : TriggerPort  TriggerType=function-call  VariantControl=Variant
  Bus Assignment1 : BusAssignment  AssignedSignals=SteerWheelAngSign,SteerWheelAng,SteerWheelSpd,SAS_Sts
  Bus Assignment2 : BusAssignment  AssignedSignals=FLWheelSpd,FRWheelSpd,RLWheelSpd,RRWheelSpd,FLWheelDriveDirection,FRWheelDriveDirection,RLWheelDriveDirection,RRWheelDriveDirection,VehStandstill
  Bus Assignment3 : BusAssignment  AssignedSignals=VehLgtAccel,VehYawRate
  Bus Creator : BusCreator  Inputs=11
  Bus Creator2 : BusCreator  Commented=on  Inputs=6
  Bus Creator3 : BusCreator  Inputs=4
  Bus Creator4 : BusCreator  Inputs=3
  Bus Selector : BusSelector  OutputSignals=DMS_NODE.DMS_FD1_MSG.DMSSts,DMS_NODE.DMS_FD1_MSG.HeadDetn,DMS_NODE.DMS_FD1_MSG.DistrctnLvl_ACC,DMS_NODE.DMS_FD1_MSG.DistrctnLvlQlty_ACC,DMS_NODE.DMS_FD1_MSG.DrowsnsLvl_ACC
  Bus Selector2 : BusSelector  OutputSignals=ESP_NODE.ESP_FD3_MSG.FLWheelSpd,ESP_NODE.ESP_FD3_MSG.FRWheelSpd,ESP_NODE.ESP_FD3_MSG.RLWheelSpd,ESP_NODE.ESP_FD3_MSG.RRWheelSpd,ESP_NODE.ESP_FD3_MSG.FLWheelDriveDirection,ESP_NODE.ESP_FD3_MSG.FRWheelDriveDirection,ESP_NODE.ESP_FD3_MSG.RLWheelDriveDirection,ESP_NODE.ESP_FD3_MSG.RRWheelDriveDirection,ESP_NODE.ESP_FD2_MSG.VehStandstill
  Bus Selector3 : BusSelector  OutputSignals=CSA_NODE.CSA2_MSG.SteerWheelAngSign,CSA_NODE.CSA2_MSG.SteerWheelAng,CSA_NODE.CSA2_MSG.SteerWheelSpd,CSA_NODE.CSA2_MSG.SAS_Sts
  Bus Selector4 : BusSelector  OutputSignals=ABM_NODE.ABM2_MSG.VehLgtAccel,ABM_NODE.ABM2_MSG.VehYawRate
  Bus Selector8 : BusSelector  Commented=on  OutputSignals=ESP_NODE.ESP_FD2_MSG.VehSpd
  CAL : Subsystem
  Constant1 : Constant  Value=0  OutDataTypeStr=Bus: VCAN_CSA_MSG_BUS
  Constant2 : Constant  Value=0  OutDataTypeStr=Bus: VCAN_ABM_MSG_BUS
  Constant3 : Constant  Value=0  OutDataTypeStr=Bus: VCAN_ESP_MSG_BUS
  DMS : ModelReference  Commented=on  ModelNameDialog=PubIfCommonDMS_MDL.slx  SimulationMode=Normal  ModelReferenceVersion=3.0
  Data Outport : dsmpblib/Data Outport  Priority=-10000  Commented=on
      settings: SourceProductName=dSPACE Model Interface Blockset
  Data Outport1 : dsmpblib/Data Outport  Priority=-10000  Commented=on
      settings: SourceProductName=dSPACE Model Interface Blockset
  EHR : ModelReference  Commented=on  ModelNameDialog=PubIfCommonEHRV2_MDL_New.slx  SimulationMode=Normal  ModelReferenceVersion=1.4
  Ground : Ground  Commented=on
  S-Function Builder : S-Function  Commented=on  FunctionName=SWC_VIE  SFunctionModules=SWC_VIE_wrapper PubIfCommonVIE_MDL  SFunctionDeploymentMode=off  EnableBusSupport=off  mask(S-Function Builder){}
      mask help: Simulink:masks:SFunctionBuilder_MD
      mask init:
      | val = [[.9  0.75 0.75 1 1 .9 .9 1]',[1 1 0.75 0.75 .9 .9 1 .9]'];try , sys = get_param(gcb,'SfunBuilderFcnName');if isempty(sys), sys = get_param(gcb,'FunctionName'); end,catch, sys = get_param(gcb,'FunctionName'); end
      settings: CopyFcn=set_param(gcbh,'LinkStatus','none')  OpenFcn=sfunctionwizard(gcbh)
      mask Display: plot(val(:,1),val(:,2)),disp(sys),port_label('input',1,'arg_VIE_VCAN_ESP'),port_label('input',2,'arg_VIE_VCAN_CSA'),port_label('input',3,'arg_VIE_VCAN_ABM'),port_label('output',1,'arg_axvRefMs2'),port_label('output',2,'arg_vxvRefMs'),port_label('output',3,'arg_axvRoadSlopeMs2'),port_label('output',4,'arg_axRefMs2'),port_label('output',5,'arg_axRefDt'),port_label('output',6,'arg_psiDtOpt'),port_label('output',7,'arg_ayvRefMs2'),port_label('output',8,'arg_alpSideSlipAngle'),port_label('output',9,'arg_kapTraj'),port_label('output',10,'arg_alpSumSlideCurveness'),port_label('output',11,'arg_SteerAngleOffset_deg')
  Subsystem1 : Subsystem  Commented=on
  Subsystem2 : Subsystem  Commented=on
  Subsystem3 : Subsystem  Commented=on
  Subsystem4 : Subsystem  Commented=on
  Subsystem5 : Subsystem  Commented=on
  Subsystem6 : Subsystem  Commented=on
  Subsystem7 : Subsystem
  VIE : ModelReference  ModelNameDialog=PubIfCommonVIE_MDL.slx  SimulationMode=Normal  ModelReferenceVersion=3.6
  IfCALBus : Outport
  IfDMSBus : Outport  Port=2
  IfVIEBus : Outport  Port=3
  IfEHRBus : Outport  Port=4
  wires:
  Bus Assignment3/1 -> VIE/3
  Bus Selector4/2 -> Bus Assignment3/3  "<VehYawRate>"
  Bus Selector4/1 -> Bus Assignment3/2  "<VehLgtAccel>"
  Constant2/1 -> Bus Assignment3/1
  Bus Assignment1/1 -> VIE/2
  Bus Selector3/4 -> Bus Assignment1/5  "<SAS_Sts>"
  Bus Selector3/3 -> Bus Assignment1/4  "<SteerWheelSpd>"
  Bus Selector3/2 -> Bus Assignment1/3  "<SteerWheelAng>"
  Bus Selector3/1 -> Bus Assignment1/2  "<SteerWheelAngSign>"
  Constant1/1 -> Bus Assignment1/1
  Bus Assignment2/1 -> VIE/1
  Bus Selector2/9 -> Bus Assignment2/10  "<VehStandstill>"
  Bus Selector2/8 -> Bus Assignment2/9  "<RRWheelDriveDirection>"
  Bus Selector2/7 -> Bus Assignment2/8  "<RLWheelDriveDirection>"
  Bus Selector2/6 -> Bus Assignment2/7  "<FRWheelDriveDirection>"
  Bus Selector2/5 -> Bus Assignment2/6  "<FLWheelDriveDirection>"
  Bus Selector2/4 -> Bus Assignment2/5  "<RRWheelSpd>"
  Bus Selector2/3 -> Bus Assignment2/4  "<RLWheelSpd>"
  Bus Selector2/2 -> Bus Assignment2/3  "<FRWheelSpd>"
  Bus Selector2/1 -> Bus Assignment2/2  "<FLWheelSpd>"
  Constant3/1 -> Bus Assignment2/1
  EHR/6 -> Bus Creator2/6  "EHRV2_DYNAMIC_INFO"
  EHR/5 -> Bus Creator2/5  "EHRV2_NAV_INFO"
  EHR/4 -> Bus Creator2/4  "EHRV2_ROAD_INFO"
  EHR/3 -> Bus Creator2/3  "EHRV2_ROAD_ROI"
  EHR/2 -> Bus Creator2/2  "EHRV2_HutHandshake"
  EHR/1 -> Bus Creator2/1  "EHRV2_HDR"
  [IfCANBus] -> Bus Selector2/1, Bus Selector3/1, Bus Selector4/1
  Bus Selector/5 -> Subsystem7/5(DrowsnsLvl_ACC)  "<DrowsnsLvl_ACC>"
  Bus Selector/4 -> Subsystem7/4(DistrctnLvlQlty_ACC)  "<DistrctnLvlQlty_ACC>"
  Bus Selector/3 -> Subsystem7/3(DistrctnLvl_ACC)  "<DistrctnLvl_ACC>"
  Bus Selector/2 -> Subsystem7/2(HeadDetn)  "<HeadDetn>"
  Bus Selector/1 -> Subsystem7/1(DMSSts)  "<DMSSts>"
  [IfCANBus] -> Subsystem1/1(In1), Subsystem5/1(In1), Subsystem3/1(In1), Subsystem2/1(In1), Subsystem4/1(In1), Subsystem6/1(In1), Bus Selector8/1
  Ground/1 -> EHR/8
  Bus Selector8/1 -> EHR/7  "<VehSpd>"
  Subsystem6/1(EHRV2_VCAN_META) -> EHR/6
  Subsystem2/1(EHRV2_VCAN_PROFSHORT) -> EHR/4
  Subsystem4/1(EHRV2_VCAN_PROFLONG) -> EHR/5
  Subsystem5/1(EHRV2_VCAN_SEG) -> EHR/2
  Subsystem3/1(EHRV2_VCAN_STUB) -> EHR/3
  Subsystem1/1(EHRV2_VCAN_POSN) -> EHR/1
  VIE/11 -> Bus Creator/11  "SteerAngleOffset_deg"
  CAL/1(CAL_VSM_CONFIG) -> Bus Creator3/1  "CAL_VSM_CONFIG"
  VIE/5 -> Bus Creator/5  "axRefDt"
  VIE/3 -> Bus Creator/3  "axvRoadSlopeMs2"
  VIE/10 -> Bus Creator/10  "alpSumSlideCurveness"
  Subsystem7/3(DMS_DriverSts) -> Bus Creator4/3  "DriverSts"
  CAL/4(CAL_AHBC_CONFIG) -> Bus Creator3/4  "CAL_AHBC_CONFIG"
  CAL/3(NvMReadWriteU8) -> Bus Creator3/3  "NvMReadWriteU8"
  VIE/7 -> Bus Creator/7  "ayvRefMs2"
  Bus Creator4/1 -> IfDMSBus/1  "IfDMSBus"
  VIE/4 -> Bus Creator/4  "axRefMs2"
  [IfCANBus] -> Bus Selector/1
  IfCANBus/1 -> [IfCANBus]
  Subsystem7/1(DMS_DistractnSts) -> Bus Creator4/1  "DistractnSts"
  Subsystem7/2(DMS_DrowsnsSts) -> Bus Creator4/2  "DrowsnsSts"
  Bus Creator2/1 -> IfEHRBus/1  "IfEHRBus"
  Bus Creator/1 -> IfVIEBus/1  "IfVIEBus"
  VIE/9 -> Bus Creator/9  "kapTraj"
  VIE/2 -> Bus Creator/2  "vxvRefMs"
  VIE/1 -> Bus Creator/1  "axvRefMs2"
  CAL/2(CAL_AEB_CONFIG) -> Bus Creator3/2  "CAL_AEB_CONFIG"
  VIE/6 -> Bus Creator/6  "psiDtOpt"
  Bus Creator3/1 -> IfCALBus/1  "IfCALBus"
  VIE/8 -> Bus Creator/8  "alpSideSlipAngle"

== system Noh_Nofusion/Control1 ==
  note: VMC-LON
      | (LongtitudeControl)
  note: VMC-LAT
      | (LateralControl)
  IfVCANBus : Inport  OutDataTypeStr=Bus: VCAN_BUS
  IfVSMBus : Inport  Port=2
  IfTOSBus : Inport  Port=3
  IfRFMBus : Inport  Port=4
  IfEHRBus : Inport  Port=5
  IfVIEBus : Inport  Port=6
  IfRoadBus : Inport  Port=7
  IfPlanbus : Inport  Port=8
  roadwidth : Inport  Port=9
  function : TriggerPort  TriggerType=function-call  VariantControl=Variant
  Bus Assignment : BusAssignment  AssignedSignals=dCurrentLaneWidth
  Bus Assignment1 : BusAssignment  AssignedSignals=CURRENT_GEAR,SHIFT_IN_PROGRESS
  Bus Assignment2 : BusAssignment  AssignedSignals=NoBrkForce,VehStandstill
  Bus Assignment4 : BusAssignment  AssignedSignals=ACU_ShiftInProgress,HCU_PTDrvMod,TotWheelTrq,MinPsblWheelTrq
  Bus Creator1 : BusCreator  Inputs=3
  Bus Creator2 : BusCreator  Inputs=4
  Bus Creator3 : BusCreator  Inputs=4
  Bus Selector : BusSelector  OutputSignals=PLAN_ACCPLAN,PLAN_Longctrl_DecelToStopReq
  Bus Selector1 : BusSelector  OutputSignals=vxvRefMs,axvRefMs2,ayvRefMs2,kapTraj,alpSideSlipAngle,psiDtOpt,SteerAngleOffset_deg
  Bus Selector11 : BusSelector  OutputSignals=RFM_ROAD
  Bus Selector13 : BusSelector  OutputSignals=DCT_NODE.DCT5_MSG.CURRENT_GEAR,DCT_NODE.DCT5_MSG.SHIFT_IN_PROGRESS
  Bus Selector2 : BusSelector  OutputSignals=EPS_NODE.EPS_FD1_MSG.EPS_SteerMod,EPS_NODE.EPS_FD1_MSG.EPS_DrvInpTrqVal_HighReslolution,EPS_NODE.EPS_FD1_MSG.EPS_LKATorqOvrlDlvd,EPS_NODE.EPS_FD1_MSG.EPS_LKATorqOvrlDlvdVld
  Bus Selector3 : BusSelector  OutputSignals=vxvRefMs,axvRoadSlopeMs2,axRefMs2,alpSideSlipAngle,axRefDt
  Bus Selector4 : BusSelector  OutputSignals=CSA_NODE.CSA2_MSG.SteerWheelAng,CSA_NODE.CSA2_MSG.SteerWheelAngSign,CSA_NODE.CSA2_MSG.SteerWheelSpd,CSA_NODE.CSA2_MSG.SteerWheelSpdSign
  Bus Selector5 : BusSelector  OutputSignals=ESP_NODE.ESP_FD2_MSG.NoBrkForce,ESP_NODE.ESP_FD2_MSG.VehStandstill
  Bus Selector6 : BusSelector  OutputSignals=VSM_LAT_CTRL
  Bus Selector7 : BusSelector  OutputSignals=HCU_NODE.HCU_FD1_MSG.ACU_ShiftInProgress,HCU_NODE.HCU_FD3_MSG.HCU_PTDrvMod,HCU_NODE.HCU_FD1_MSG.TotWheelTrq,HCU_NODE.HCU_FD1_MSG.MinPsblWheelTrq
  Bus Selector8 : BusSelector  OutputSignals=VSM_LON_CTRL
  Bus Creator : BusCreator  Inputs=4
  Constant1 : Constant  Value=0  OutDataTypeStr=Bus: VCAN_DCT_MSG_BUS
  Constant3 : Constant  Value=0  OutDataTypeStr=Bus: VCAN_ESP_MSG_BUS
  Constant4 : Constant  Value=0  OutDataTypeStr=Bus: VCAN_HCU_MSG_BUS
  Data Type Conversion : DataTypeConversion
  LATC : ModelReference  ModelNameDialog=PubIfControlLATC_MDL.slx  SimulationMode=Normal  ModelReferenceVersion=3.279
  LON : ModelReference  ModelNameDialog=PubIfControlLONC_MDL.slx  SimulationMode=Normal  ModelReferenceVersion=3.54
  Signal Copy : SignalConversion  OverrideOpt=off
  Subsystem : Subsystem
  Terminator : Terminator
  Terminator2 : Terminator
  IfLONBus : Outport
  IfLATBus : Outport  Port=2
  wires:
  Signal Copy/1 -> LATC/6
  Bus Creator/1 -> IfLATBus/1
  roadwidth/1 -> Data Type Conversion/1, [roadwidth]
  Bus Assignment/1 -> LATC/11
  Data Type Conversion/1 -> Bus Assignment/2
  Bus Selector7/4 -> Bus Assignment4/5  "<MinPsblWheelTrq>"
  Bus Selector7/2 -> Bus Assignment4/3  "<HCU_PTDrvMod>"
  Bus Selector7/3 -> Bus Assignment4/4  "<TotWheelTrq>"
  Bus Selector7/1 -> Bus Assignment4/2  "<ACU_ShiftInProgress>"
  Bus Assignment4/1 -> LON/9
  Subsystem/1(Out1) -> LON/8
  Constant4/1 -> Bus Assignment4/1
  Bus Assignment1/1 -> LON/7
  Bus Selector13/2 -> Bus Assignment1/3  "<SHIFT_IN_PROGRESS>"
  Bus Selector13/1 -> Bus Assignment1/2  "<CURRENT_GEAR>"
  Constant1/1 -> Bus Assignment1/1
  Bus Selector5/2 -> Bus Assignment2/3  "<VehStandstill>"
  Bus Selector5/1 -> Bus Assignment2/2  "<NoBrkForce>"
  Bus Assignment2/1 -> LON/6
  Constant3/1 -> Bus Assignment2/1
  Bus Selector/2 -> LON/12  "<PLAN_Longctrl_DecelToStopReq>"
  IfTOSBus/1 -> Terminator2/1
  IfRFMBus/1 -> Terminator/1
  Bus Selector/1 -> LON/11  "<PLAN_ACCPLAN>"
  Bus Selector8/1 -> LON/10  "<VSM_LON_CTRL>"
  Bus Selector3/5 -> LON/5  "<axRefDt>"
  Bus Selector3/4 -> LON/4  "<alpSideSlipAngle>"
  Bus Selector3/3 -> LON/3  "<axRefMs2>"
  Bus Selector3/2 -> LON/2  "<axvRoadSlopeMs2>"
  Bus Selector3/1 -> LON/1  "<vxvRefMs>"
  IfPlanbus/1 -> Bus Selector/1
  Bus Selector1/6 -> LATC/7  "<psiDtOpt>"
  Bus Selector1/5 -> Signal Copy/1  "<alpSideSlipAngle>"
  Bus Selector1/4 -> LATC/5  "<kapTraj>"
  Bus Selector1/3 -> LATC/4  "<ayvRefMs2>"
  Bus Selector1/2 -> LATC/3  "<axvRefMs2>"
  Bus Selector1/1 -> LATC/2  "<vxvRefMs>"
  Bus Selector6/1 -> LATC/1  "<VSM_LAT_CTRL>"
  Bus Creator3/1 -> LATC/10
  Bus Selector4/4 -> Bus Creator3/4  "<SteerWheelSpdSign>"
  Bus Selector4/1 -> Bus Creator3/1  "<SteerWheelAng>"
  Bus Selector4/3 -> Bus Creator3/3  "<SteerWheelSpd>"
  Bus Selector4/2 -> Bus Creator3/2  "<SteerWheelAngSign>"
  Bus Creator2/1 -> LATC/9
  Bus Selector2/1 -> Bus Creator2/1  "<EPS_SteerMod>"
  Bus Selector2/4 -> Bus Creator2/4  "<EPS_LKATorqOvrlDlvdVld>"
  Bus Selector2/2 -> Bus Creator2/2  "<EPS_DrvInpTrqVal_HighReslolution>"
  Bus Selector2/3 -> Bus Creator2/3  "<EPS_LKATorqOvrlDlvd>"
  Bus Selector1/7 -> LATC/8  "<SteerAngleOffset_deg>"
  Bus Selector11/1 -> Bus Assignment/1  "<RFM_ROAD>"
  IfRoadBus/1 -> Bus Selector11/1
  IfVSMBus/1 -> Bus Selector6/1, Bus Selector8/1
  IfVCANBus/1 -> Bus Selector2/1, Bus Selector4/1, Bus Selector5/1, Bus Selector13/1, Subsystem/1(In1), Bus Selector7/1
  Bus Creator1/1 -> IfLONBus/1  "IfLONBus"
  IfVIEBus/1 -> Bus Selector1/1, Bus Selector3/1
  LATC/1 -> Bus Creator/1  "IFCTrqOvlCmdReqValue"
  LATC/2 -> Bus Creator/2  "IFCFuncTrqCmdReqFlag"
  LATC/3 -> Bus Creator/3  "LATC_IFCFuncAngCmdReqFlag"
  LATC/4 -> Bus Creator/4  "LATC_IFCAngCmdReqValue"
  LON/1 -> Bus Creator1/1  "LONC_CTRL_OUT"
  LON/2 -> Bus Creator1/2  "LONC_Hybrid_CTRL_OUT"
  LON/3 -> Bus Creator1/3  "LONC_VLC_InternalAcc"
